simulink model "PID"  (R2023a)
settings: Solver=VariableStepAuto  StartTime=0.0  StopTime=1000  RelTol=1e-3
PreLoadFcn:
  | eta = Simulink.Signal;
  | eta.CoderInfo.StorageClass = 'ExportedGlobal';
  | eta.InitialValue = '[0 0 0 0 0 0]';
  | V = Simulink.Signal;
  | V.CoderInfo.StorageClass = 'ExportedGlobal';
  | V.InitialValue = '[0 0 0 0 0 0]';
model workspace: external: MATLAB File /home/ponbapanda/study_material/ee4901/6DOF-UUV/src/OdeRexRov.m (data not in the file)
values from neighbouring files (symbols this model uses):
  M = MRB + MA    [ModelRexRov.m]
  Minv = inv(M)    [FeedLin.m]
libraries: slpidlib x6, simulink x2
settings Model: Creator=ponbapanda  LastModifiedBy=ponbapanda

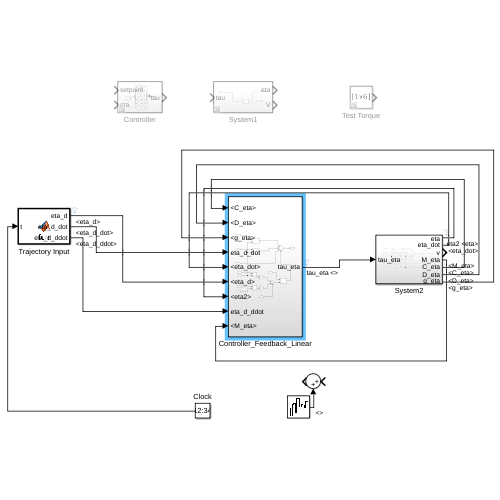
[thumbnail: Simulink's stored preview of the top-level diagram]
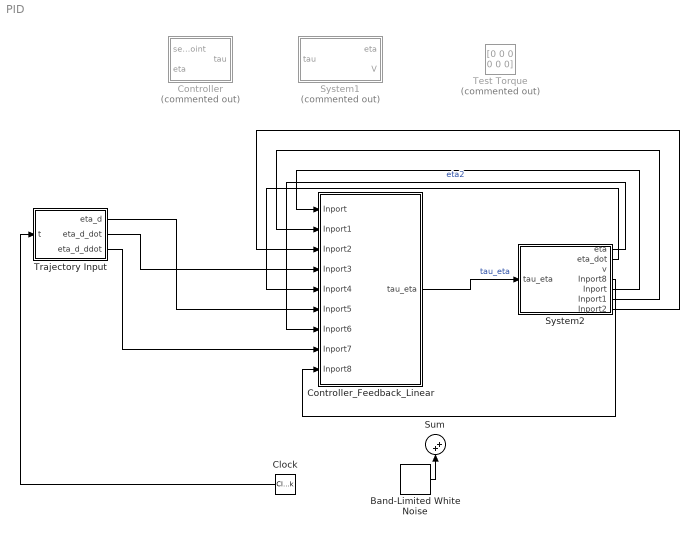
== system PID ==
  Band-Limited White Noise : simulink/Sources/Band-Limited White Noise  Cov=[0.00001 0.00001 0.00001 0.0005 0.0005 0.0005]  Ts=0.05  seed=[23341]
  Clock : DigitalClock  SampleTime=0.05
  Controller : Subsystem  Commented=on
  Controller_Feedback_Linear : Subsystem
  Sum : Sum  Inputs=|++
  System1 : Subsystem  Commented=on
  System2 : Subsystem
  Test Torque : Constant  Commented=on  Value=[0 0 0 0 0 0]
  Trajectory Input : MATLAB Function  TreatAsAtomicUnit=on
  wires:
  Clock/1 -> Trajectory Input/1(t)
  Band-Limited White Noise/1 -> Sum/2
  System2/4(Inport8) -> Controller_Feedback_Linear/9(Inport8)
  System2/5(Inport) -> Controller_Feedback_Linear/1(Inport)
  System2/6(Inport1) -> Controller_Feedback_Linear/2(Inport1)
  System2/7(Inport2) -> Controller_Feedback_Linear/3(Inport2)
  System2/1(eta) -> Controller_Feedback_Linear/7(Inport6)  "eta2"
  System2/2(eta_dot) -> Controller_Feedback_Linear/5(Inport4)
  Trajectory Input/1(eta_d) -> Controller_Feedback_Linear/6(Inport5)
  Controller_Feedback_Linear/1(tau_eta) -> System2/1(tau_eta)  "tau_eta"
  Trajectory Input/2(eta_d_dot) -> Controller_Feedback_Linear/4(Inport3)
  Trajectory Input/3(eta_d_ddot) -> Controller_Feedback_Linear/8(Inport7)

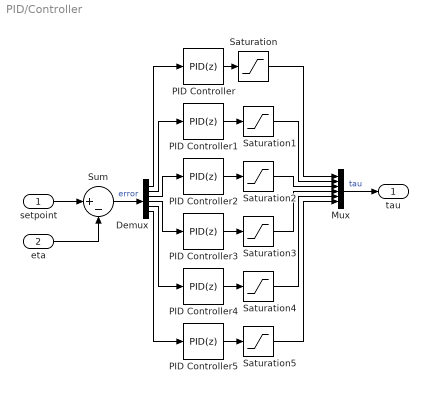
== system PID/Controller ==
  setpoint : Inport
  eta : Inport  Port=2
  Demux : Demux  Outputs=6
  Mux : Mux  Inputs=6
  PID Controller : slpidlib/PID Controller  Controller=PID  Form=Parallel  TimeDomain=Discrete-time  UseExternalTs=off  SampleTime=0.0500000000000000028  IntegratorMethod=Forward Euler  FilterMethod=Forward Euler  ControllerParametersSource=internal  P=500.000000000000000  I=10.000000000000000  UseKiTs=off  D=503.391827453152189  N=19.865241060018288  UseFilter=on  TunerSelectOption=Transfer Function Based (PID Tuner App)  InitialConditionSource=internal  InitialConditionForIntegrator=0  InitialConditionForFilter=0  DifferentiatorICPrevScaledInput=0  ExternalReset=none  TrackingMode=off  Kt=1  LimitOutput=off  SatLimitsSource=internal  UpperSaturationLimit=inf  LowerSaturationLimit=-inf  LinearizeAsGain=on  AntiWindupMode=none  Kb=1  LimitIntegrator=off  UpperIntegratorSaturationLimit=inf  LowerIntegratorSaturationLimit=-inf  POutMin=[]  POutMax=[]  IOutMin=[]  IOutMax=[]  DOutMin=[]  DOutMax=[]  NOutMin=[]  NOutMax=[]  SumOutMin=[]  SumOutMax=[]  SaturationOutMin=[]  SaturationOutMax=[]  PParamMin=[]  PParamMax=[]  IParamMin=[]  IParamMax=[]  DParamMin=[]  DParamMax=[]  NParamMin=[]  NParamMax=[]  KbParamMin=[]  KbParamMax=[]  KtParamMin=[]  KtParamMax=[]  KbOutMin=[]  KbOutMax=[]  KtOutMin=[]  KtOutMax=[]  IntegratorOutMin=[]  IntegratorOutMax=[]  FilterOutMin=[]  FilterOutMax=[]  SumI1OutMin=[]  SumI1OutMax=[]  SumI2OutMin=[]  SumI2OutMax=[]  SumI3OutMin=[]  SumI3OutMax=[]  SumI4OutMin=[]  SumI4OutMax=[]  SumDOutMin=[]  SumDOutMax=[]  DifferentiatorOutMin=[]  DifferentiatorOutMax=[]  FilterDiffOutCoefMin=[]  FilterDiffOutCoefMax=[]  ReciprocalOutMin=[]  ReciprocalOutMax=[]  SumDenOutMin=[]  SumDenOutMax=[]  SumNumOutMin=[]  SumNumOutMax=[]  DivideOutMin=[]  DivideOutMax=[]  UdiffTsProdOutMin=[]  UdiffTsProdOutMax=[]  NTsProdOutMin=[]  NTsProdOutMax=[]  UintegralTsProdOutMin=[]  UintegralTsProdOutMax=[]  UngainTsProdOutMin=[]  UngainTsProdOutMax=[]  ClampingZeroOutDataTypeStr=Inherit: Inherit via back propagation  ClampingZeroOutMin=[]  ClampingZeroOutMax=[]  FilterDenConstantOutDataTypeStr=Inherit: Inherit via back propagation  FilterDenConstantOutMin=[]  FilterDenConstantOutMax=[]  PCopyOutDataTypeStr=Inherit: Inherit via back propagation  PCopyOutMin=[]  PCopyOutMax=[]  NCopyOutDataTypeStr=Inherit: Inherit via back propagation  NCopyOutMin=[]  NCopyOutMax=[]  IntegratorContinuousStateAttributes=''  IntegratorStateMustResolveToSignalObject=off  IntegratorRTWStateStorageClass=Auto  FilterContinuousStateAttributes=''  FilterStateMustResolveToSignalObject=off  FilterRTWStateStorageClass=Auto  ParallelPVariant=InternalParameters  IdealPVariant=Disabled  IVariant=InternalParameters  DVariant=InternalParameters  IntegratorVariant=Discrete  SatVariant=Disabled  AWVariant=Passthrough  PCopyVariant=Disabled  TRVariant=Disabled  FdbkBlocksVariant=Forward  IdealPFdbkVariant=Disabled  SatFdbkVariant=Disabled  DerivativeFilterVariant=ForwardEulerFilter  NVariant=InternalParameters  NCopyVariant=Disabled  FilterICVariant=InternalICsFilter  IntegratorICVariant=InternalICs  ExternalResetVariant=Disabled  TRSumVariant=Passthrough  SumFdbkVariant=Disabled  SumVariant=Sum_PID  TsampFilterVariant=InternalTs  TsampNgainVariant=Passthrough  TsampIntegralVariant=Disabled_SignalSpec  ExternalSaturationOutDataTypeStr=Inherit: Same as second input
  PID Controller1 : slpidlib/PID Controller  Controller=PID  Form=Parallel  TimeDomain=Discrete-time  UseExternalTs=off  SampleTime=0.0500000000000000028  IntegratorMethod=Forward Euler  FilterMethod=Forward Euler  ControllerParametersSource=internal  P=500.000000000000000  I=10.000000000000000  UseKiTs=off  D=503.391827453152189  N=19.865241060018288  UseFilter=on  TunerSelectOption=Transfer Function Based (PID Tuner App)  InitialConditionSource=internal  InitialConditionForIntegrator=0  InitialConditionForFilter=0  DifferentiatorICPrevScaledInput=0  ExternalReset=none  TrackingMode=off  Kt=1  LimitOutput=off  SatLimitsSource=internal  UpperSaturationLimit=inf  LowerSaturationLimit=-inf  LinearizeAsGain=on  AntiWindupMode=none  Kb=1  LimitIntegrator=off  UpperIntegratorSaturationLimit=inf  LowerIntegratorSaturationLimit=-inf  POutMin=[]  POutMax=[]  IOutMin=[]  IOutMax=[]  DOutMin=[]  DOutMax=[]  NOutMin=[]  NOutMax=[]  SumOutMin=[]  SumOutMax=[]  SaturationOutMin=[]  SaturationOutMax=[]  PParamMin=[]  PParamMax=[]  IParamMin=[]  IParamMax=[]  DParamMin=[]  DParamMax=[]  NParamMin=[]  NParamMax=[]  KbParamMin=[]  KbParamMax=[]  KtParamMin=[]  KtParamMax=[]  KbOutMin=[]  KbOutMax=[]  KtOutMin=[]  KtOutMax=[]  IntegratorOutMin=[]  IntegratorOutMax=[]  FilterOutMin=[]  FilterOutMax=[]  SumI1OutMin=[]  SumI1OutMax=[]  SumI2OutMin=[]  SumI2OutMax=[]  SumI3OutMin=[]  SumI3OutMax=[]  SumI4OutMin=[]  SumI4OutMax=[]  SumDOutMin=[]  SumDOutMax=[]  DifferentiatorOutMin=[]  DifferentiatorOutMax=[]  FilterDiffOutCoefMin=[]  FilterDiffOutCoefMax=[]  ReciprocalOutMin=[]  ReciprocalOutMax=[]  SumDenOutMin=[]  SumDenOutMax=[]  SumNumOutMin=[]  SumNumOutMax=[]  DivideOutMin=[]  DivideOutMax=[]  UdiffTsProdOutMin=[]  UdiffTsProdOutMax=[]  NTsProdOutMin=[]  NTsProdOutMax=[]  UintegralTsProdOutMin=[]  UintegralTsProdOutMax=[]  UngainTsProdOutMin=[]  UngainTsProdOutMax=[]  ClampingZeroOutDataTypeStr=Inherit: Inherit via back propagation  ClampingZeroOutMin=[]  ClampingZeroOutMax=[]  FilterDenConstantOutDataTypeStr=Inherit: Inherit via back propagation  FilterDenConstantOutMin=[]  FilterDenConstantOutMax=[]  PCopyOutDataTypeStr=Inherit: Inherit via back propagation  PCopyOutMin=[]  PCopyOutMax=[]  NCopyOutDataTypeStr=Inherit: Inherit via back propagation  NCopyOutMin=[]  NCopyOutMax=[]  IntegratorContinuousStateAttributes=''  IntegratorStateMustResolveToSignalObject=off  IntegratorRTWStateStorageClass=Auto  FilterContinuousStateAttributes=''  FilterStateMustResolveToSignalObject=off  FilterRTWStateStorageClass=Auto  ParallelPVariant=InternalParameters  IdealPVariant=Disabled  IVariant=InternalParameters  DVariant=InternalParameters  IntegratorVariant=Discrete  SatVariant=Disabled  AWVariant=Passthrough  PCopyVariant=Disabled  TRVariant=Disabled  FdbkBlocksVariant=Forward  IdealPFdbkVariant=Disabled  SatFdbkVariant=Disabled  DerivativeFilterVariant=ForwardEulerFilter  NVariant=InternalParameters  NCopyVariant=Disabled  FilterICVariant=InternalICsFilter  IntegratorICVariant=InternalICs  ExternalResetVariant=Disabled  TRSumVariant=Passthrough  SumFdbkVariant=Disabled  SumVariant=Sum_PID  TsampFilterVariant=InternalTs  TsampNgainVariant=Passthrough  TsampIntegralVariant=Disabled_SignalSpec  ExternalSaturationOutDataTypeStr=Inherit: Same as second input
  PID Controller2 : slpidlib/PID Controller  Controller=PID  Form=Parallel  TimeDomain=Discrete-time  UseExternalTs=off  SampleTime=0.0500000000000000028  IntegratorMethod=Forward Euler  FilterMethod=Forward Euler  ControllerParametersSource=internal  P=500.000000000000000  I=0.000000000000000  UseKiTs=off  D=503.391827453152189  N=19.865241060018288  UseFilter=on  TunerSelectOption=Transfer Function Based (PID Tuner App)  InitialConditionSource=internal  InitialConditionForIntegrator=0  InitialConditionForFilter=0  DifferentiatorICPrevScaledInput=0  ExternalReset=none  TrackingMode=off  Kt=1  LimitOutput=off  SatLimitsSource=internal  UpperSaturationLimit=inf  LowerSaturationLimit=-inf  LinearizeAsGain=on  AntiWindupMode=none  Kb=1  LimitIntegrator=off  UpperIntegratorSaturationLimit=inf  LowerIntegratorSaturationLimit=-inf  POutMin=[]  POutMax=[]  IOutMin=[]  IOutMax=[]  DOutMin=[]  DOutMax=[]  NOutMin=[]  NOutMax=[]  SumOutMin=[]  SumOutMax=[]  SaturationOutMin=[]  SaturationOutMax=[]  PParamMin=[]  PParamMax=[]  IParamMin=[]  IParamMax=[]  DParamMin=[]  DParamMax=[]  NParamMin=[]  NParamMax=[]  KbParamMin=[]  KbParamMax=[]  KtParamMin=[]  KtParamMax=[]  KbOutMin=[]  KbOutMax=[]  KtOutMin=[]  KtOutMax=[]  IntegratorOutMin=[]  IntegratorOutMax=[]  FilterOutMin=[]  FilterOutMax=[]  SumI1OutMin=[]  SumI1OutMax=[]  SumI2OutMin=[]  SumI2OutMax=[]  SumI3OutMin=[]  SumI3OutMax=[]  SumI4OutMin=[]  SumI4OutMax=[]  SumDOutMin=[]  SumDOutMax=[]  DifferentiatorOutMin=[]  DifferentiatorOutMax=[]  FilterDiffOutCoefMin=[]  FilterDiffOutCoefMax=[]  ReciprocalOutMin=[]  ReciprocalOutMax=[]  SumDenOutMin=[]  SumDenOutMax=[]  SumNumOutMin=[]  SumNumOutMax=[]  DivideOutMin=[]  DivideOutMax=[]  UdiffTsProdOutMin=[]  UdiffTsProdOutMax=[]  NTsProdOutMin=[]  NTsProdOutMax=[]  UintegralTsProdOutMin=[]  UintegralTsProdOutMax=[]  UngainTsProdOutMin=[]  UngainTsProdOutMax=[]  ClampingZeroOutDataTypeStr=Inherit: Inherit via back propagation  ClampingZeroOutMin=[]  ClampingZeroOutMax=[]  FilterDenConstantOutDataTypeStr=Inherit: Inherit via back propagation  FilterDenConstantOutMin=[]  FilterDenConstantOutMax=[]  PCopyOutDataTypeStr=Inherit: Inherit via back propagation  PCopyOutMin=[]  PCopyOutMax=[]  NCopyOutDataTypeStr=Inherit: Inherit via back propagation  NCopyOutMin=[]  NCopyOutMax=[]  IntegratorContinuousStateAttributes=''  IntegratorStateMustResolveToSignalObject=off  IntegratorRTWStateStorageClass=Auto  FilterContinuousStateAttributes=''  FilterStateMustResolveToSignalObject=off  FilterRTWStateStorageClass=Auto  ParallelPVariant=InternalParameters  IdealPVariant=Disabled  IVariant=InternalParameters  DVariant=InternalParameters  IntegratorVariant=Discrete  SatVariant=Disabled  AWVariant=Passthrough  PCopyVariant=Disabled  TRVariant=Disabled  FdbkBlocksVariant=Forward  IdealPFdbkVariant=Disabled  SatFdbkVariant=Disabled  DerivativeFilterVariant=ForwardEulerFilter  NVariant=InternalParameters  NCopyVariant=Disabled  FilterICVariant=InternalICsFilter  IntegratorICVariant=InternalICs  ExternalResetVariant=Disabled  TRSumVariant=Passthrough  SumFdbkVariant=Disabled  SumVariant=Sum_PID  TsampFilterVariant=InternalTs  TsampNgainVariant=Passthrough  TsampIntegralVariant=Disabled_SignalSpec  ExternalSaturationOutDataTypeStr=Inherit: Same as second input
  PID Controller3 : slpidlib/PID Controller  Controller=PID  Form=Parallel  TimeDomain=Discrete-time  UseExternalTs=off  SampleTime=0.0500000000000000028  IntegratorMethod=Forward Euler  FilterMethod=Forward Euler  ControllerParametersSource=internal  P=5000.000000000000000  I=500.000000000000000  UseKiTs=off  D=503.391827453152189  N=19.865241060018288  UseFilter=on  TunerSelectOption=Transfer Function Based (PID Tuner App)  InitialConditionSource=internal  InitialConditionForIntegrator=0  InitialConditionForFilter=0  DifferentiatorICPrevScaledInput=0  ExternalReset=none  TrackingMode=off  Kt=1  LimitOutput=off  SatLimitsSource=internal  UpperSaturationLimit=inf  LowerSaturationLimit=-inf  LinearizeAsGain=on  AntiWindupMode=none  Kb=1  LimitIntegrator=off  UpperIntegratorSaturationLimit=inf  LowerIntegratorSaturationLimit=-inf  POutMin=[]  POutMax=[]  IOutMin=[]  IOutMax=[]  DOutMin=[]  DOutMax=[]  NOutMin=[]  NOutMax=[]  SumOutMin=[]  SumOutMax=[]  SaturationOutMin=[]  SaturationOutMax=[]  PParamMin=[]  PParamMax=[]  IParamMin=[]  IParamMax=[]  DParamMin=[]  DParamMax=[]  NParamMin=[]  NParamMax=[]  KbParamMin=[]  KbParamMax=[]  KtParamMin=[]  KtParamMax=[]  KbOutMin=[]  KbOutMax=[]  KtOutMin=[]  KtOutMax=[]  IntegratorOutMin=[]  IntegratorOutMax=[]  FilterOutMin=[]  FilterOutMax=[]  SumI1OutMin=[]  SumI1OutMax=[]  SumI2OutMin=[]  SumI2OutMax=[]  SumI3OutMin=[]  SumI3OutMax=[]  SumI4OutMin=[]  SumI4OutMax=[]  SumDOutMin=[]  SumDOutMax=[]  DifferentiatorOutMin=[]  DifferentiatorOutMax=[]  FilterDiffOutCoefMin=[]  FilterDiffOutCoefMax=[]  ReciprocalOutMin=[]  ReciprocalOutMax=[]  SumDenOutMin=[]  SumDenOutMax=[]  SumNumOutMin=[]  SumNumOutMax=[]  DivideOutMin=[]  DivideOutMax=[]  UdiffTsProdOutMin=[]  UdiffTsProdOutMax=[]  NTsProdOutMin=[]  NTsProdOutMax=[]  UintegralTsProdOutMin=[]  UintegralTsProdOutMax=[]  UngainTsProdOutMin=[]  UngainTsProdOutMax=[]  ClampingZeroOutDataTypeStr=Inherit: Inherit via back propagation  ClampingZeroOutMin=[]  ClampingZeroOutMax=[]  FilterDenConstantOutDataTypeStr=Inherit: Inherit via back propagation  FilterDenConstantOutMin=[]  FilterDenConstantOutMax=[]  PCopyOutDataTypeStr=Inherit: Inherit via back propagation  PCopyOutMin=[]  PCopyOutMax=[]  NCopyOutDataTypeStr=Inherit: Inherit via back propagation  NCopyOutMin=[]  NCopyOutMax=[]  IntegratorContinuousStateAttributes=''  IntegratorStateMustResolveToSignalObject=off  IntegratorRTWStateStorageClass=Auto  FilterContinuousStateAttributes=''  FilterStateMustResolveToSignalObject=off  FilterRTWStateStorageClass=Auto  ParallelPVariant=InternalParameters  IdealPVariant=Disabled  IVariant=InternalParameters  DVariant=InternalParameters  IntegratorVariant=Discrete  SatVariant=Disabled  AWVariant=Passthrough  PCopyVariant=Disabled  TRVariant=Disabled  FdbkBlocksVariant=Forward  IdealPFdbkVariant=Disabled  SatFdbkVariant=Disabled  DerivativeFilterVariant=ForwardEulerFilter  NVariant=InternalParameters  NCopyVariant=Disabled  FilterICVariant=InternalICsFilter  IntegratorICVariant=InternalICs  ExternalResetVariant=Disabled  TRSumVariant=Passthrough  SumFdbkVariant=Disabled  SumVariant=Sum_PID  TsampFilterVariant=InternalTs  TsampNgainVariant=Passthrough  TsampIntegralVariant=Disabled_SignalSpec  ExternalSaturationOutDataTypeStr=Inherit: Same as second input
  PID Controller4 : slpidlib/PID Controller  Controller=PID  Form=Parallel  TimeDomain=Discrete-time  UseExternalTs=off  SampleTime=0.0500000000000000028  IntegratorMethod=Forward Euler  FilterMethod=Forward Euler  ControllerParametersSource=internal  P=5000.000000000000000  I=500.000000000000000  UseKiTs=off  D=503.391827453152189  N=19.865241060018288  UseFilter=on  TunerSelectOption=Transfer Function Based (PID Tuner App)  InitialConditionSource=internal  InitialConditionForIntegrator=0  InitialConditionForFilter=0  DifferentiatorICPrevScaledInput=0  ExternalReset=none  TrackingMode=off  Kt=1  LimitOutput=off  SatLimitsSource=internal  UpperSaturationLimit=inf  LowerSaturationLimit=-inf  LinearizeAsGain=on  AntiWindupMode=none  Kb=1  LimitIntegrator=off  UpperIntegratorSaturationLimit=inf  LowerIntegratorSaturationLimit=-inf  POutMin=[]  POutMax=[]  IOutMin=[]  IOutMax=[]  DOutMin=[]  DOutMax=[]  NOutMin=[]  NOutMax=[]  SumOutMin=[]  SumOutMax=[]  SaturationOutMin=[]  SaturationOutMax=[]  PParamMin=[]  PParamMax=[]  IParamMin=[]  IParamMax=[]  DParamMin=[]  DParamMax=[]  NParamMin=[]  NParamMax=[]  KbParamMin=[]  KbParamMax=[]  KtParamMin=[]  KtParamMax=[]  KbOutMin=[]  KbOutMax=[]  KtOutMin=[]  KtOutMax=[]  IntegratorOutMin=[]  IntegratorOutMax=[]  FilterOutMin=[]  FilterOutMax=[]  SumI1OutMin=[]  SumI1OutMax=[]  SumI2OutMin=[]  SumI2OutMax=[]  SumI3OutMin=[]  SumI3OutMax=[]  SumI4OutMin=[]  SumI4OutMax=[]  SumDOutMin=[]  SumDOutMax=[]  DifferentiatorOutMin=[]  DifferentiatorOutMax=[]  FilterDiffOutCoefMin=[]  FilterDiffOutCoefMax=[]  ReciprocalOutMin=[]  ReciprocalOutMax=[]  SumDenOutMin=[]  SumDenOutMax=[]  SumNumOutMin=[]  SumNumOutMax=[]  DivideOutMin=[]  DivideOutMax=[]  UdiffTsProdOutMin=[]  UdiffTsProdOutMax=[]  NTsProdOutMin=[]  NTsProdOutMax=[]  UintegralTsProdOutMin=[]  UintegralTsProdOutMax=[]  UngainTsProdOutMin=[]  UngainTsProdOutMax=[]  ClampingZeroOutDataTypeStr=Inherit: Inherit via back propagation  ClampingZeroOutMin=[]  ClampingZeroOutMax=[]  FilterDenConstantOutDataTypeStr=Inherit: Inherit via back propagation  FilterDenConstantOutMin=[]  FilterDenConstantOutMax=[]  PCopyOutDataTypeStr=Inherit: Inherit via back propagation  PCopyOutMin=[]  PCopyOutMax=[]  NCopyOutDataTypeStr=Inherit: Inherit via back propagation  NCopyOutMin=[]  NCopyOutMax=[]  IntegratorContinuousStateAttributes=''  IntegratorStateMustResolveToSignalObject=off  IntegratorRTWStateStorageClass=Auto  FilterContinuousStateAttributes=''  FilterStateMustResolveToSignalObject=off  FilterRTWStateStorageClass=Auto  ParallelPVariant=InternalParameters  IdealPVariant=Disabled  IVariant=InternalParameters  DVariant=InternalParameters  IntegratorVariant=Discrete  SatVariant=Disabled  AWVariant=Passthrough  PCopyVariant=Disabled  TRVariant=Disabled  FdbkBlocksVariant=Forward  IdealPFdbkVariant=Disabled  SatFdbkVariant=Disabled  DerivativeFilterVariant=ForwardEulerFilter  NVariant=InternalParameters  NCopyVariant=Disabled  FilterICVariant=InternalICsFilter  IntegratorICVariant=InternalICs  ExternalResetVariant=Disabled  TRSumVariant=Passthrough  SumFdbkVariant=Disabled  SumVariant=Sum_PID  TsampFilterVariant=InternalTs  TsampNgainVariant=Passthrough  TsampIntegralVariant=Disabled_SignalSpec  ExternalSaturationOutDataTypeStr=Inherit: Same as second input
  PID Controller5 : slpidlib/PID Controller  Controller=PID  Form=Parallel  TimeDomain=Discrete-time  UseExternalTs=off  SampleTime=0.0500000000000000028  IntegratorMethod=Forward Euler  FilterMethod=Forward Euler  ControllerParametersSource=internal  P=5000.000000000000000  I=500.000000000000000  UseKiTs=off  D=503.391827453152189  N=19.865241060018288  UseFilter=on  TunerSelectOption=Transfer Function Based (PID Tuner App)  InitialConditionSource=internal  InitialConditionForIntegrator=0  InitialConditionForFilter=0  DifferentiatorICPrevScaledInput=0  ExternalReset=none  TrackingMode=off  Kt=1  LimitOutput=off  SatLimitsSource=internal  UpperSaturationLimit=inf  LowerSaturationLimit=-inf  LinearizeAsGain=on  AntiWindupMode=none  Kb=1  LimitIntegrator=off  UpperIntegratorSaturationLimit=inf  LowerIntegratorSaturationLimit=-inf  POutMin=[]  POutMax=[]  IOutMin=[]  IOutMax=[]  DOutMin=[]  DOutMax=[]  NOutMin=[]  NOutMax=[]  SumOutMin=[]  SumOutMax=[]  SaturationOutMin=[]  SaturationOutMax=[]  PParamMin=[]  PParamMax=[]  IParamMin=[]  IParamMax=[]  DParamMin=[]  DParamMax=[]  NParamMin=[]  NParamMax=[]  KbParamMin=[]  KbParamMax=[]  KtParamMin=[]  KtParamMax=[]  KbOutMin=[]  KbOutMax=[]  KtOutMin=[]  KtOutMax=[]  IntegratorOutMin=[]  IntegratorOutMax=[]  FilterOutMin=[]  FilterOutMax=[]  SumI1OutMin=[]  SumI1OutMax=[]  SumI2OutMin=[]  SumI2OutMax=[]  SumI3OutMin=[]  SumI3OutMax=[]  SumI4OutMin=[]  SumI4OutMax=[]  SumDOutMin=[]  SumDOutMax=[]  DifferentiatorOutMin=[]  DifferentiatorOutMax=[]  FilterDiffOutCoefMin=[]  FilterDiffOutCoefMax=[]  ReciprocalOutMin=[]  ReciprocalOutMax=[]  SumDenOutMin=[]  SumDenOutMax=[]  SumNumOutMin=[]  SumNumOutMax=[]  DivideOutMin=[]  DivideOutMax=[]  UdiffTsProdOutMin=[]  UdiffTsProdOutMax=[]  NTsProdOutMin=[]  NTsProdOutMax=[]  UintegralTsProdOutMin=[]  UintegralTsProdOutMax=[]  UngainTsProdOutMin=[]  UngainTsProdOutMax=[]  ClampingZeroOutDataTypeStr=Inherit: Inherit via back propagation  ClampingZeroOutMin=[]  ClampingZeroOutMax=[]  FilterDenConstantOutDataTypeStr=Inherit: Inherit via back propagation  FilterDenConstantOutMin=[]  FilterDenConstantOutMax=[]  PCopyOutDataTypeStr=Inherit: Inherit via back propagation  PCopyOutMin=[]  PCopyOutMax=[]  NCopyOutDataTypeStr=Inherit: Inherit via back propagation  NCopyOutMin=[]  NCopyOutMax=[]  IntegratorContinuousStateAttributes=''  IntegratorStateMustResolveToSignalObject=off  IntegratorRTWStateStorageClass=Auto  FilterContinuousStateAttributes=''  FilterStateMustResolveToSignalObject=off  FilterRTWStateStorageClass=Auto  ParallelPVariant=InternalParameters  IdealPVariant=Disabled  IVariant=InternalParameters  DVariant=InternalParameters  IntegratorVariant=Discrete  SatVariant=Disabled  AWVariant=Passthrough  PCopyVariant=Disabled  TRVariant=Disabled  FdbkBlocksVariant=Forward  IdealPFdbkVariant=Disabled  SatFdbkVariant=Disabled  DerivativeFilterVariant=ForwardEulerFilter  NVariant=InternalParameters  NCopyVariant=Disabled  FilterICVariant=InternalICsFilter  IntegratorICVariant=InternalICs  ExternalResetVariant=Disabled  TRSumVariant=Passthrough  SumFdbkVariant=Disabled  SumVariant=Sum_PID  TsampFilterVariant=InternalTs  TsampNgainVariant=Passthrough  TsampIntegralVariant=Disabled_SignalSpec  ExternalSaturationOutDataTypeStr=Inherit: Same as second input
  Saturation : Saturate  UpperLimit=8000  LowerLimit=-8000  LinearizeAsGain=off  ZeroCross=off
  Saturation1 : Saturate  UpperLimit=8000  LowerLimit=-8000  LinearizeAsGain=off  ZeroCross=off
  Saturation2 : Saturate  UpperLimit=8000  LowerLimit=-8000  LinearizeAsGain=off  ZeroCross=off
  Saturation3 : Saturate  UpperLimit=100000  LowerLimit=-100000  LinearizeAsGain=off  ZeroCross=off
  Saturation4 : Saturate  UpperLimit=100000  LowerLimit=-100000  LinearizeAsGain=off  ZeroCross=off
  Saturation5 : Saturate  UpperLimit=100000  LowerLimit=-100000  LinearizeAsGain=off  ZeroCross=off
  Sum : Sum  Inputs=|+-
  tau : Outport
  wires:
  PID Controller5/1 -> Saturation5/1
  setpoint/1 -> Sum/1
  PID Controller1/1 -> Saturation1/1
  Mux/1 -> tau/1  "tau"
  Saturation4/1 -> Mux/5
  Saturation/1 -> Mux/1
  Demux/5 -> PID Controller4/1
  eta/1 -> Sum/2
  PID Controller3/1 -> Saturation3/1
  Demux/2 -> PID Controller1/1
  Demux/4 -> PID Controller3/1
  Saturation2/1 -> Mux/3
  Demux/3 -> PID Controller2/1
  Demux/6 -> PID Controller5/1
  Saturation5/1 -> Mux/6
  Saturation3/1 -> Mux/4
  PID Controller2/1 -> Saturation2/1
  Sum/1 -> Demux/1  "error"
  Saturation1/1 -> Mux/2
  Demux/1 -> PID Controller/1
  PID Controller/1 -> Saturation/1
  PID Controller4/1 -> Saturation4/1

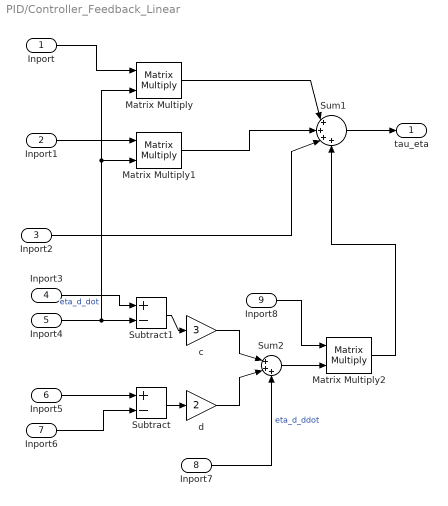
== system PID/Controller_Feedback_Linear ==
  Inport : Inport
  Inport1 : Inport  Port=2
  Inport2 : Inport  Port=3
  Inport3 : Inport  Port=4
  Inport4 : Inport  Port=5
  Inport5 : Inport  Port=6
  Inport6 : Inport  Port=7
  Inport7 : Inport  Port=8
  Inport8 : Inport  Port=9
  Matrix Multiply : Product  Multiplication=Matrix(*)
  Matrix Multiply1 : Product  Multiplication=Matrix(*)
  Matrix Multiply2 : Product  Multiplication=Matrix(*)
  Subtract : Sum  Inputs=+-
  Subtract1 : Sum  Inputs=+-
  Sum1 : Sum  Inputs=|++++
  Sum2 : Sum  Inputs=|+++
  c : Gain  Gain=3
  d : Gain  Gain=2
  tau_eta : Outport
  wires:
  Inport7/1 -> Sum2/3  "eta_d_ddot"
  c/1 -> Sum2/1
  Inport3/1 -> Subtract1/1  "eta_d_dot"
  Matrix Multiply1/1 -> Sum1/2
  Inport/1 -> Matrix Multiply/1
  Matrix Multiply2/1 -> Sum1/4
  Inport4/1 -> Subtract1/2, Matrix Multiply/2, Matrix Multiply1/2
  Sum2/1 -> Matrix Multiply2/2
  d/1 -> Sum2/2
  Sum1/1 -> tau_eta/1
  Inport1/1 -> Matrix Multiply1/1
  Inport6/1 -> Subtract/2
  Inport5/1 -> Subtract/1
  Inport8/1 -> Matrix Multiply2/1
  Subtract1/1 -> c/1
  Inport2/1 -> Sum1/3
  Subtract/1 -> d/1
  Matrix Multiply/1 -> Sum1/1

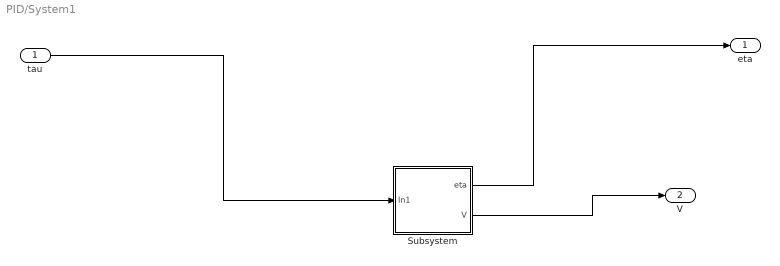
== system PID/System1 ==
  tau : Inport
  Subsystem : Subsystem
  eta : Outport
  V : Outport  Port=2
  wires:
  tau/1 -> Subsystem/1(In1)
  Subsystem/1(eta) -> eta/1
  Subsystem/2(V) -> V/1

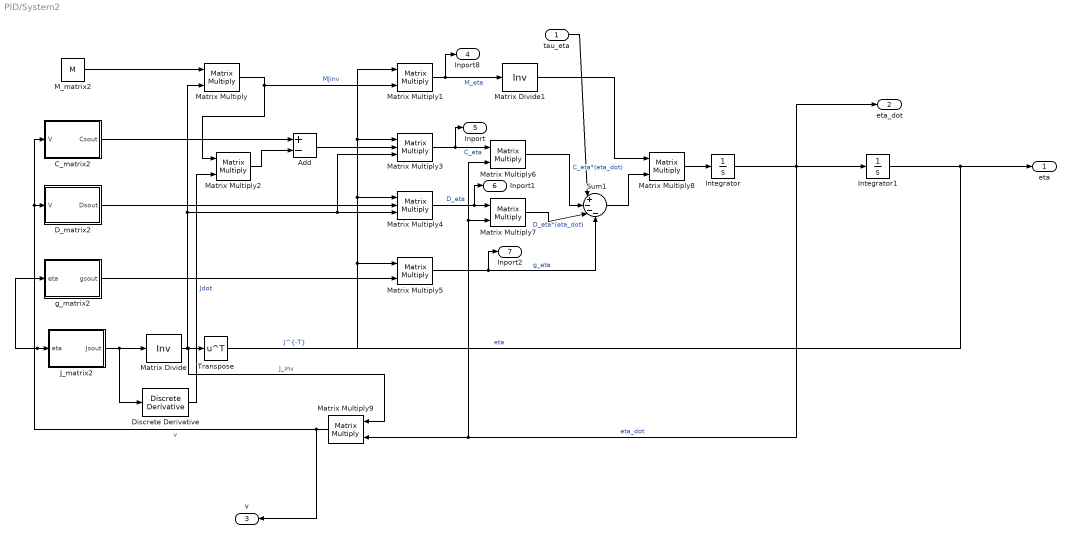
== system PID/System2 ==
  tau_eta : Inport
  Add : Sum  Inputs=+-
  C_matrix2 : MATLAB Function  TreatAsAtomicUnit=on
  D_matrix2 : MATLAB Function  TreatAsAtomicUnit=on
  Discrete Derivative : simulink/Discrete/Discrete Derivative  gainval=1.0  ICPrevScaledInput=0.0  OutMin=[]  OutMax=[]  OutDataType=fixdt(1, 16)  OutScaling=2^-10  DoSatur=off
  Integrator : Integrator  InitialCondition=[0,0,0,0,0,0].'
  Integrator1 : Integrator  InitialCondition=[0 0 0 0 0 0].'
  J_matrix2 : MATLAB Function  TreatAsAtomicUnit=on
  M_matrix2 : Constant  Value=M
  Matrix Divide : Product  Inputs=/  Multiplication=Matrix(*)
  Matrix Divide1 : Product  Inputs=/  Multiplication=Matrix(*)
  Matrix Multiply{,1..2,5..9} (8 alike) : Product  Multiplication=Matrix(*)
  Matrix Multiply3 : Product  Inputs=3  Multiplication=Matrix(*)
  Matrix Multiply4 : Product  Inputs=3  Multiplication=Matrix(*)
  Sum1 : Sum  Inputs=|+---
  Transpose : Math  Operator=transpose
  g_matrix2 : MATLAB Function  TreatAsAtomicUnit=on
  eta : Outport
  eta_dot : Outport  Port=2
  v : Outport  Port=3
  Inport8 : Outport  Port=4
  Inport : Outport  Port=5
  Inport1 : Outport  Port=6
  Inport2 : Outport  Port=7
  wires:
  tau_eta/1 -> Sum1/1
  Add/1 -> Matrix Multiply3/2
  Matrix Multiply3/1 -> Inport/1, Matrix Multiply6/1  "C_eta"
  D_matrix2/1(Dsout) -> Matrix Multiply4/2
  g_matrix2/1(gsout) -> Matrix Multiply5/2
  Matrix Multiply2/1 -> Add/2
  Sum1/1 -> Matrix Multiply8/2
  Matrix Multiply5/1 -> Inport2/1, Sum1/4  "g_eta"
  Matrix Divide/1 -> Matrix Multiply9/1, Transpose/1, Matrix Multiply/2, Matrix Multiply3/3, Matrix Multiply4/3  "J_inv"
  Matrix Multiply7/1 -> Sum1/3  "D_eta*(eta_dot)"
  Matrix Multiply6/1 -> Sum1/2  "C_eta*(eta_dot)"
  J_matrix2/1(Jsout) -> Discrete Derivative/1, Matrix Divide/1
  Matrix Multiply9/1 -> v/1, C_matrix2/1(V), D_matrix2/1(V)  "v"
  Matrix Divide1/1 -> Matrix Multiply8/1
  Transpose/1 -> Matrix Multiply5/1, Matrix Multiply1/1, Matrix Multiply3/1, Matrix Multiply4/1  "J^{-T}"
  Matrix Multiply1/1 -> Inport8/1, Matrix Divide1/1  "M_eta"
  Matrix Multiply/1 -> Matrix Multiply2/1, Matrix Multiply1/2  "MJinv"
  M_matrix2/1 -> Matrix Multiply/1
  Matrix Multiply8/1 -> Integrator/1
  Discrete Derivative/1 -> Matrix Multiply2/2  "Jdot"
  Matrix Multiply4/1 -> Inport1/1, Matrix Multiply7/1  "D_eta"
  C_matrix2/1(Csout) -> Add/1
  Integrator/1 -> Matrix Multiply7/2, Matrix Multiply6/2, Matrix Multiply9/2, Integrator1/1, eta_dot/1  "eta_dot"
  Integrator1/1 -> eta/1, g_matrix2/1(eta), J_matrix2/1(eta)  "eta"

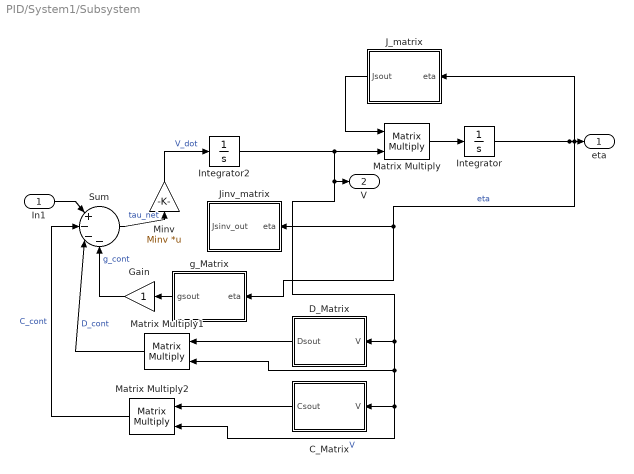
== system PID/System1/Subsystem ==
  In1 : Inport
  C_Matrix : MATLAB Function  TreatAsAtomicUnit=on
  D_Matrix : MATLAB Function  TreatAsAtomicUnit=on
  Gain : Gain
  Integrator : Integrator  InitialCondition=[5 0 0 0 0 pi]
  Integrator2 : Integrator  InitialCondition=[5 0 0 0 0 0]
  J_matrix : MATLAB Function  TreatAsAtomicUnit=on
  Jinv_matrix : MATLAB Function  TreatAsAtomicUnit=on
  Matrix Multiply : Product  Multiplication=Matrix(*)
  Matrix Multiply1 : Product  Multiplication=Matrix(*)
  Matrix Multiply2 : Product  Multiplication=Matrix(*)
  Minv : Gain  Gain=Minv  Multiplication=Matrix(K*u) (u vector)
  Sum : Sum  Inputs=|+---
  g_Matrix : MATLAB Function  TreatAsAtomicUnit=on
  eta : Outport
  V : Outport  Port=2
  wires:
  J_matrix/1(Jsout) -> Matrix Multiply/1
  Matrix Multiply1/1 -> Sum/3  "D_cont"
  Matrix Multiply2/1 -> Sum/2  "C_cont"
  D_Matrix/1(Dsout) -> Matrix Multiply1/1
  C_Matrix/1(Csout) -> Matrix Multiply2/1
  Matrix Multiply/1 -> Integrator/1
  Gain/1 -> Sum/4  "g_cont"
  Minv/1 -> Integrator2/1  "V_dot"
  In1/1 -> Sum/1
  Integrator/1 -> J_matrix/1(eta), g_Matrix/1(eta), Jinv_matrix/1(eta), eta/1  "eta"
  Integrator2/1 -> Matrix Multiply1/2, C_Matrix/1(V), Matrix Multiply2/2, D_Matrix/1(V), V/1, Matrix Multiply/2  "V"
  Sum/1 -> Minv/1  "tau_net"
  g_Matrix/1(gsout) -> Gain/1

== matlab function PID/System1/Subsystem/J_matrix ==
  data: eta input; Jsout output
function Jsout = Js(eta)
x = eta(1,:);
y = eta(2,:);
z = eta(3,:);
phi = eta(4,:);
theta = eta(5,:);
psi = eta(6,:);
t2 = cos(phi);
t3 = cos(psi);
t4 = cos(theta);
t5 = sin(phi);
t6 = sin(psi);
t7 = sin(theta);
t8 = tan(theta);
t9 = 1.0./t4;
Jsout = reshape([t3.*t4,t4.*t6,t7.*-1.0,0.0,0.0,0.0,t2.*t6.*-1.0+t3.*t5.*t7,t2.*t3+t5.*t6.*t7,t4.*t5,0.0,0.0,0.0,t5.*t6+t2.*t3.*t7,t3.*t5.*-1.0+t2.*t6.*t7,t2.*t4,0.0,0.0,0.0,0.0,0.0,0.0,1.0,0.0,0.0,0.0,0.0,0.0,t5.*t8,t2,t5.*t9,0.0,0.0,0.0,t2.*t8,t5.*-1.0,t2.*t9],[6,6]);
end

== matlab function PID/System1/Subsystem/D_Matrix ==
  data: V input; Dsout output
function Dsout = Ds(V)
u = V(1,:);
v = V(2,:);
w = V(3,:);
p = V(4,:);
q = V(5,:);
r = V(6,:);
Dsout = reshape([abs(u).*7.4822e+2+7.482e+1,0.0,0.0,0.0,0.0,0.0,0.0,abs(v).*9.9253e+2+6.948e+1,0.0,0.0,0.0,0.0,0.0,0.0,abs(w).*1.82101e+3+7.284e+2,0.0,0.0,0.0,0.0,0.0,0.0,abs(p).*6.72e+2+2.688e+2,0.0,0.0,0.0,0.0,0.0,0.0,abs(q).*7.7444e+2+3.0977e+2,0.0,0.0,0.0,0.0,0.0,0.0,abs(r).*5.2327e+2+1.05e+2],[6,6]);

== matlab function PID/System1/Subsystem/C_Matrix ==
  data: V input; Csout output
function Csout = Cs(V)
u = V(1,:);
v = V(2,:);
w = V(3,:);
p = V(4,:);
q = V(5,:);
r = V(6,:);
t2 = p.*1.060290000000037e+3;
t3 = p.*-8.542600000000675;
t4 = p.*8.542600000000675;
t5 = p.*8.586999999999989;
t6 = q.*8.586999999999989;
t7 = u.*8.542600000000675;
t8 = q.*-1.655400000000081e+2;
t9 = q.*1.655400000000081e+2;
t10 = u.*-2.642660000000149e+3;
t11 = u.*2.642660000000149e+3;
t12 = u.*1.655400000000081e+2;
t13 = r.*-1.077399999999943e+1;
t14 = r.*1.077399999999943e+1;
t15 = w.*1.077499999999964e+1;
t16 = w.*-5.522770000000019e+3;
t17 = w.*5.522770000000019e+3;
t18 = q.*-5.848799999999756;
t19 = q.*5.848799999999756;
t20 = q.*1.483799999999974;
t21 = r.*1.483799999999974;
t22 = q.*-3.864199999999837e+2;
t23 = q.*3.864199999999837e+2;
t24 = p.*-6.111200000000281;
t25 = p.*6.111200000000281;
t26 = v.*5.848799999999756;
t27 = p.*-4.094400000000023e+2;
t28 = p.*4.094400000000023e+2;
t29 = v.*-3.084870000000112e+3;
t30 = v.*3.084870000000112e+3;
t31 = q.*1.636889999999898e+3;
t32 = w.*3.864199999999837e+2;
t33 = w.*6.111200000000281;
t34 = u.*-1.03320000000007e+2;
t35 = u.*1.03320000000007e+2;
t36 = v.*4.094400000000023e+2;
t37 = v.*-5.129000000000087e+1;
t38 = v.*5.129000000000087e+1;
t39 = p.*5.442900000000373e+1;
t40 = w.*-5.129000000000087e+1;
t41 = w.*5.129000000000087e+1;
t42 = w.*-1.03320000000007e+2;
t43 = w.*1.03320000000007e+2;
t44 = r.*5.442900000000373e+1;
t45 = u.*-6.877300000000105;
t46 = u.*6.877300000000105;
t47 = v.*-6.877300000000105;
t48 = v.*6.877300000000105;
t49 = r.*9.155499999999884e+2;
t50 = r.*-7.803299999999581;
t51 = r.*7.803299999999581;
t52 = r.*-6.272600000000239e+1;
t53 = r.*6.272600000000239e+1;
t54 = u.*7.803299999999581;
t55 = v.*6.272600000000239e+1;
t56 = t3+t9+t10+t43+t48+t51;
t57 = t4+t8+t11+t42+t47+t50;
t58 = t13+t16+t23+t24+t35+t37;
t59 = t14+t17+t22+t25+t34+t38;
t60 = t19+t27+t29+t40+t46+t52;
t61 = t18+t28+t30+t41+t45+t53;
Csout = reshape([0.0,0.0,0.0,0.0,t58,t61,0.0,0.0,0.0,t59,0.0,t56,0.0,0.0,0.0,t60,t57,0.0,0.0,t58,t61,0.0,-t15-t20-t39-t49+t54-t55,-t5-t12+t21-t26+t31-t32,t59,0.0,t56,t15+t20+t39+t49-t54+t55,0.0,-t2+t6-t7-t33-t36-t44,t60,t57,0.0,t5+t12-t21+t26-t31+t32,t2-t6+t7+t33+t36+t44,0.0],[6,6]);
end

== matlab function PID/System1/Subsystem/Jinv_matrix ==
  data: eta input; Jsinv_out output
function Jsinv_out = Jsinv(eta)

x = eta(1,:);
y = eta(2,:);
z = eta(3,:);
phi = eta(4,:);
theta = eta(5,:);
psi = eta(6,:);
t2 = cos(phi);
t3 = cos(psi);
t4 = cos(theta);
t5 = sin(phi);
t6 = sin(psi);
t7 = sin(theta);
t8 = t2.^2;
t9 = t3.^2;
t10 = t4.^2;
t11 = t5.^2;
t12 = t6.^2;
t13 = t7.^2;
t14 = t8.*t10;
t15 = t9.*t10;
t16 = t8+t11;
t17 = t8.*t13;
t18 = t10.*t11;
t19 = t9.*t13;
t20 = t10.*t12;
t21 = t11.*t13;
t22 = t12.*t13;
t23 = 1.0./t16;
t24 = t9.*t17;
t25 = t12.*t14;
t26 = t11.*t15;
t27 = t12.*t17;
t28 = t11.*t19;
t29 = t12.*t18;
t30 = t12.*t21;
t31 = t9.*t14;
t32 = t14+t17+t18+t21;
t33 = t15+t19+t20+t22;
t34 = 1.0./t32;
t35 = 1.0./t33;
t36 = t24+t25+t26+t27+t28+t29+t30+t31;
t37 = 1.0./t36;
Jsinv_out = reshape([t3.*t4.*t35.*1.0,t37.*(t3.*t5.*t7.*-1.0+t2.*t6.*t10+t2.*t6.*t13).*-1.0,t37.*(t2.*t3.*t7+t5.*t6.*t10+t5.*t6.*t13).*1.0,0.0,0.0,0.0,t4.*t6.*t35.*1.0,t37.*(t2.*t3.*t10+t2.*t3.*t13+t5.*t6.*t7).*1.0,t37.*(-t2.*t6.*t7+t3.*t5.*t10.*1.0+t3.*t5.*t13.*1.0).*-1.0,0.0,0.0,0.0,(t7.*-1.0)./(t10+t13),t4.*t5.*t34.*1.0,t2.*t4.*t34.*1.0,0.0,0.0,0.0,0.0,0.0,0.0,1.0,0.0,0.0,0.0,0.0,0.0,0.0,t2.*t23.*1.0,t5.*t23.*-1.0,0.0,0.0,0.0,t4.*tan(theta).*-1.0,t4.*t5.*t23.*1.0,t2.*t4.*t23.*1.0],[6,6]);
end

== matlab function PID/Trajectory Input ==
  data: t input; eta_d output; eta_d_dot output; eta_d_ddot output
function [eta_d,eta_d_dot,eta_d_ddot]= fcn(t)
%if t>400
%    setpoint = [0.05*(t-400);0;0;0;0;0];
%elseif t>200
%    setpoint = [0.05*(400-t);0;0;0;0;0];
%else
%    setpoint = [0.05*t;0;0;0;0;0];
eta_d = [5*sin(t);0;0;0;0;t];
eta_d_dot = [5*cos(t);0;0;0;0;1];
eta_d_ddot = [-5*sin(t);0;0;0;0;0];
%setpoint = [0;0.5*sin(t/10);0;0;0;0];
%setpoint = [0.5*cos(t/10);0.5*sin(t/10);0;0;0;0];
%setpoint = [0;0;0;1.5*sin(t/10);0;0];
%setpoint = [0;0;0;0;0;0.5*sin(t/10)];
%setpoint = [3*t;0;0;0;0.52*sin(t);0];
%setpoint = [0;0;0;0;0;0.05*t];
%eta_d = [0;0;0;0;0;0];
end

== matlab function PID/System2/C_matrix2 ==
  data: V input; Csout output
function Csout = Cs(V)
u = V(1,:);
v = V(2,:);
w = V(3,:);
p = V(4,:);
q = V(5,:);
r = V(6,:);
t2 = p.*1.060290000000037e+3;
t3 = p.*-8.542600000000675;
t4 = p.*8.542600000000675;
t5 = p.*8.586999999999989;
t6 = q.*8.586999999999989;
t7 = u.*8.542600000000675;
t8 = q.*-1.655400000000081e+2;
t9 = q.*1.655400000000081e+2;
t10 = u.*-2.642660000000149e+3;
t11 = u.*2.642660000000149e+3;
t12 = u.*1.655400000000081e+2;
t13 = r.*-1.077399999999943e+1;
t14 = r.*1.077399999999943e+1;
t15 = w.*1.077499999999964e+1;
t16 = w.*-5.522770000000019e+3;
t17 = w.*5.522770000000019e+3;
t18 = q.*-5.848799999999756;
t19 = q.*5.848799999999756;
t20 = q.*1.483799999999974;
t21 = r.*1.483799999999974;
t22 = q.*-3.864199999999837e+2;
t23 = q.*3.864199999999837e+2;
t24 = p.*-6.111200000000281;
t25 = p.*6.111200000000281;
t26 = v.*5.848799999999756;
t27 = p.*-4.094400000000023e+2;
t28 = p.*4.094400000000023e+2;
t29 = v.*-3.084870000000112e+3;
t30 = v.*3.084870000000112e+3;
t31 = q.*1.636889999999898e+3;
t32 = w.*3.864199999999837e+2;
t33 = w.*6.111200000000281;
t34 = u.*-1.03320000000007e+2;
t35 = u.*1.03320000000007e+2;
t36 = v.*4.094400000000023e+2;
t37 = v.*-5.129000000000087e+1;
t38 = v.*5.129000000000087e+1;
t39 = p.*5.442900000000373e+1;
t40 = w.*-5.129000000000087e+1;
t41 = w.*5.129000000000087e+1;
t42 = w.*-1.03320000000007e+2;
t43 = w.*1.03320000000007e+2;
t44 = r.*5.442900000000373e+1;
t45 = u.*-6.877300000000105;
t46 = u.*6.877300000000105;
t47 = v.*-6.877300000000105;
t48 = v.*6.877300000000105;
t49 = r.*9.155499999999884e+2;
t50 = r.*-7.803299999999581;
t51 = r.*7.803299999999581;
t52 = r.*-6.272600000000239e+1;
t53 = r.*6.272600000000239e+1;
t54 = u.*7.803299999999581;
t55 = v.*6.272600000000239e+1;
t56 = t3+t9+t10+t43+t48+t51;
t57 = t4+t8+t11+t42+t47+t50;
t58 = t13+t16+t23+t24+t35+t37;
t59 = t14+t17+t22+t25+t34+t38;
t60 = t19+t27+t29+t40+t46+t52;
t61 = t18+t28+t30+t41+t45+t53;
Csout = reshape([0.0,0.0,0.0,0.0,t58,t61,0.0,0.0,0.0,t59,0.0,t56,0.0,0.0,0.0,t60,t57,0.0,0.0,t58,t61,0.0,-t15-t20-t39-t49+t54-t55,-t5-t12+t21-t26+t31-t32,t59,0.0,t56,t15+t20+t39+t49-t54+t55,0.0,-t2+t6-t7-t33-t36-t44,t60,t57,0.0,t5+t12-t21+t26-t31+t32,t2-t6+t7+t33+t36+t44,0.0],[6,6]);
end

== matlab function PID/System2/D_matrix2 ==
  data: V input; Dsout output
function Dsout = Ds(V)
u = V(1,:);
v = V(2,:);
w = V(3,:);
p = V(4,:);
q = V(5,:);
r = V(6,:);
Dsout = reshape([abs(u).*7.4822e+2+7.482e+1,0.0,0.0,0.0,0.0,0.0,0.0,abs(v).*9.9253e+2+6.948e+1,0.0,0.0,0.0,0.0,0.0,0.0,abs(w).*1.82101e+3+7.284e+2,0.0,0.0,0.0,0.0,0.0,0.0,abs(p).*6.72e+2+2.688e+2,0.0,0.0,0.0,0.0,0.0,0.0,abs(q).*7.7444e+2+3.0977e+2,0.0,0.0,0.0,0.0,0.0,0.0,abs(r).*5.2327e+2+1.05e+2],[6,6]);

== matlab function PID/System2/g_matrix2 ==
  data: eta input; gsout output
function gsout = gs(eta)
x = eta(1,:);
y = eta(2,:);
z = eta(3,:);
phi = eta(4,:);
theta = eta(5,:);
psi = eta(6,:);
t2 = cos(phi);
t3 = cos(theta);
t4 = sin(phi);
t5 = sin(theta);
gsout = [t5.*-2.094180000000051e+2;t3.*t4.*2.094180000000051e+2;t2.*t3.*2.094180000000051e+2;t2.*t3.*-1.423280935999937e+2+t3.*t4.*7.157069849600084e+3;t5.*7.157069849600084e+3-t2.*t3.*1.51939860960003e+3;t5.*-1.423280935999937e+2+t3.*t4.*1.51939860960003e+3];
end

== matlab function PID/System2/J_matrix2 ==
  data: eta input; Jsout output
function Jsout = Js(eta)
x = eta(1,:);
y = eta(2,:);
z = eta(3,:);
phi = eta(4,:);
theta = eta(5,:);
psi = eta(6,:);
t2 = cos(phi);
t3 = cos(psi);
t4 = cos(theta);
t5 = sin(phi);
t6 = sin(psi);
t7 = sin(theta);
t8 = tan(theta);
t9 = 1.0./t4;
Jsout = reshape([t3.*t4,t4.*t6,t7.*-1.0,0.0,0.0,0.0,t2.*t6.*-1.0+t3.*t5.*t7,t2.*t3+t5.*t6.*t7,t4.*t5,0.0,0.0,0.0,t5.*t6+t2.*t3.*t7,t3.*t5.*-1.0+t2.*t6.*t7,t2.*t4,0.0,0.0,0.0,0.0,0.0,0.0,1.0,0.0,0.0,0.0,0.0,0.0,t5.*t8,t2,t5.*t9,0.0,0.0,0.0,t2.*t8,t5.*-1.0,t2.*t9],[6,6]);
end

== matlab function PID/System1/Subsystem/g_Matrix ==
  data: eta input; gsout output
function gsout = gs(eta)
x = eta(1,:);
y = eta(2,:);
z = eta(3,:);
phi = eta(4,:);
theta = eta(5,:);
psi = eta(6,:);
t2 = cos(phi);
t3 = cos(theta);
t4 = sin(phi);
t5 = sin(theta);
gsout = [t5.*-2.094180000000051e+2;t3.*t4.*2.094180000000051e+2;t2.*t3.*2.094180000000051e+2;t2.*t3.*-1.423280935999937e+2+t3.*t4.*7.157069849600084e+3;t5.*7.157069849600084e+3-t2.*t3.*1.51939860960003e+3;t5.*-1.423280935999937e+2+t3.*t4.*1.51939860960003e+3];
end
